simulink model "HubDepotModel_debug"  (Simulink 7.9)
settings: Solver=VariableStepDiscrete  StartTime=0.0  StopTime=100.0  RelTol=1e-3
libraries: simeventslib x2
settings Model: Creator=tsprock3  LastModifiedBy=tsprock3
settings DebuggingCC: SimStateOlderReleaseMsg=warning

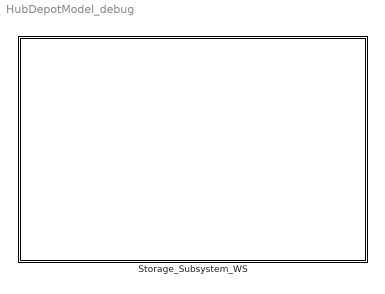
== system HubDepotModel_debug ==
  Storage_Subsystem_WS : Subsystem  AncestorBlock=DELS_Library/Storage_Subsystem_WS

== system HubDepotModel_debug/Storage_Subsystem_WS ==
  note: The Storage Subsystem mediates between the SOURCE and DELIVER channels, and provides higher levels control to those functions
  note: On the left hand side, customer procurement orders and replenishment shipments
      | come into the deliver and source functions respectively
  note: The processes associated with performing customer-facing order management and order fulfillment activities.
  note: The process of establishing and maintaining physical inventories and inventory information.
  note: The processes associated with ordering, delivery, receipt and transfer of raw material items, subassemblies, product and/or services.
  note: On the right hand side, procurement orders and fulfillment shipments
      | leave the source and deliver functions respectively
  note: The replenishment signal is primarily a mechanism for the reordering process to know that the inventory levels have
      | changed and that the inventory policy should be reviewed to determine if a procurement order is necessary. This is
      | effectively a continuous review policy
      |
      | There are other ways to accomplish this, and a periodic review policy is one such way.
  note: The INVENTORY IN/OUT is the passing of physical/electronic inventory records from their storage place in ENABLE
      |  to the functions that use the records to fulfill or procure inventory
  <<DELIVER>>Deliver_Stocked_Product : Subsystem
  <<ENABLE>> Manage_Product_Inventory : Subsystem
  <<SOURCE>> Source_Stocked_Product : Subsystem
  Customer_Procurement_Order : PMIOPort  Port=1  Side=Right
  Fulfillment_Shipment : PMIOPort  Port=2  Side=Right
  Procurement_Order : PMIOPort  Port=3  Side=Left
  Replenishment_Shipment : PMIOPort  Port=4  Side=Left
  connections:
  <<DELIVER>>Deliver_Stocked_Product/LConn2 -- Customer_Procurement_Order/RConn1
  <<DELIVER>>Deliver_Stocked_Product/RConn2 -- Fulfillment_Shipment/RConn1
  Replenishment_Shipment/RConn1 -- <<SOURCE>> Source_Stocked_Product/LConn2
  <<ENABLE>> Manage_Product_Inventory/LConn2 -- <<SOURCE>> Source_Stocked_Product/RConn1
  <<ENABLE>> Manage_Product_Inventory/RConn2 -- <<SOURCE>> Source_Stocked_Product/LConn1
  <<ENABLE>> Manage_Product_Inventory/LConn3 -- <<DELIVER>>Deliver_Stocked_Product/RConn3
  <<ENABLE>> Manage_Product_Inventory/RConn3 -- <<SOURCE>> Source_Stocked_Product/LConn3
  <<SOURCE>> Source_Stocked_Product/RConn2 -- Procurement_Order/RConn1
  <<DELIVER>>Deliver_Stocked_Product/RConn1 -- <<ENABLE>> Manage_Product_Inventory/LConn1
  <<DELIVER>>Deliver_Stocked_Product/LConn1 -- <<ENABLE>> Manage_Product_Inventory/RConn1

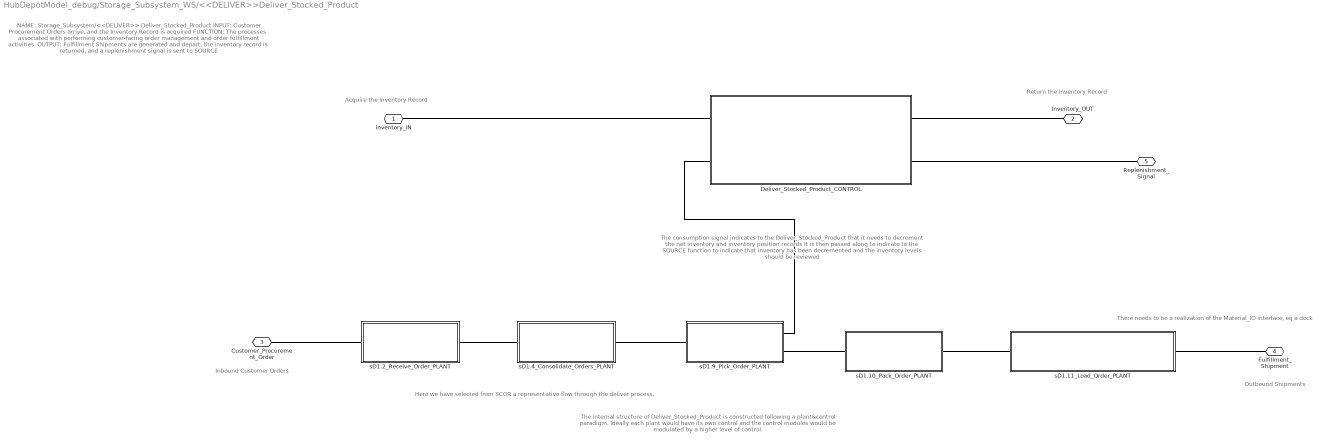
== system HubDepotModel_debug/Storage_Subsystem_WS/<<DELIVER>>Deliver_Stocked_Product ==
  note: The internal structure of Deliver_Stocked_Product is constructed following a plant&control paradigm. Ideally each plant would have its own control and the control modules would be modulated by a higher level of control.
  note: The consumption signal indicates to the Deliver_Stocked_Product that it needs to decrement the net inventory and inventory position records
      | It is then passed along to indicate to the SOURCE function to indicate that inventory has been decremented and the inventory levels should be reviewed
  note: Here we have selected from SCOR a representative flow through the deliver process.
  note: NAME: Storage_Subsystem/<<DELIVER>> Deliver_Stocked_Product
      | INPUT: Customer Procurement Orders arrive, and the Inventory Record is acquired
      | FUNCTION: The processes associated with performing customer-facing order management and order fulfillment activities.
      | OUTPUT: Fulfillment Shipments are generated and depart, the inventory record is returned, and a replenishment signal is sent to SOURCE
  note: Acquire the Inventory Record
  note: Return the Inventory Record
  note: Inbound Customer Orders
  note: Outbound Shipments
  note: There needs to be a realization of the Material_IO interface, eg a dock
  Deliver_Stocked_Product_CONTROL : Subsystem
  sD1.10_Pack_Order_PLANT : Subsystem
  sD1.11_Load_Order_PLANT : Subsystem
  sD1.2_Receive_Order_PLANT : Subsystem
  sD1.4_Consolidate_Orders_PLANT : Subsystem
  sD1.9_Pick_Order_PLANT : Subsystem
  Inventory_IN : PMIOPort  Port=1  Side=Left
  Inventory_OUT : PMIOPort  Port=2  Side=Right
  Customer_Procurement_Order : PMIOPort  Port=3  Side=Left
  Fulfillment_Shipment : PMIOPort  Port=4  Side=Right
  Replenishment_Signal : PMIOPort  Port=5  Side=Right
  connections:
  Customer_Procurement_Order/RConn1 -- sD1.2_Receive_Order_PLANT/LConn1
  sD1.9_Pick_Order_PLANT/RConn2 -- sD1.10_Pack_Order_PLANT/LConn1
  sD1.10_Pack_Order_PLANT/RConn1 -- sD1.11_Load_Order_PLANT/LConn1
  sD1.11_Load_Order_PLANT/RConn1 -- Fulfillment_Shipment/RConn1
  sD1.9_Pick_Order_PLANT/RConn1 -- Deliver_Stocked_Product_CONTROL/LConn2
  Deliver_Stocked_Product_CONTROL/LConn1 -- Inventory_IN/RConn1
  Deliver_Stocked_Product_CONTROL/RConn1 -- Inventory_OUT/RConn1
  sD1.2_Receive_Order_PLANT/RConn1 -- sD1.4_Consolidate_Orders_PLANT/LConn1
  sD1.4_Consolidate_Orders_PLANT/RConn1 -- sD1.9_Pick_Order_PLANT/LConn1
  Deliver_Stocked_Product_CONTROL/RConn2 -- Replenishment_Signal/RConn1

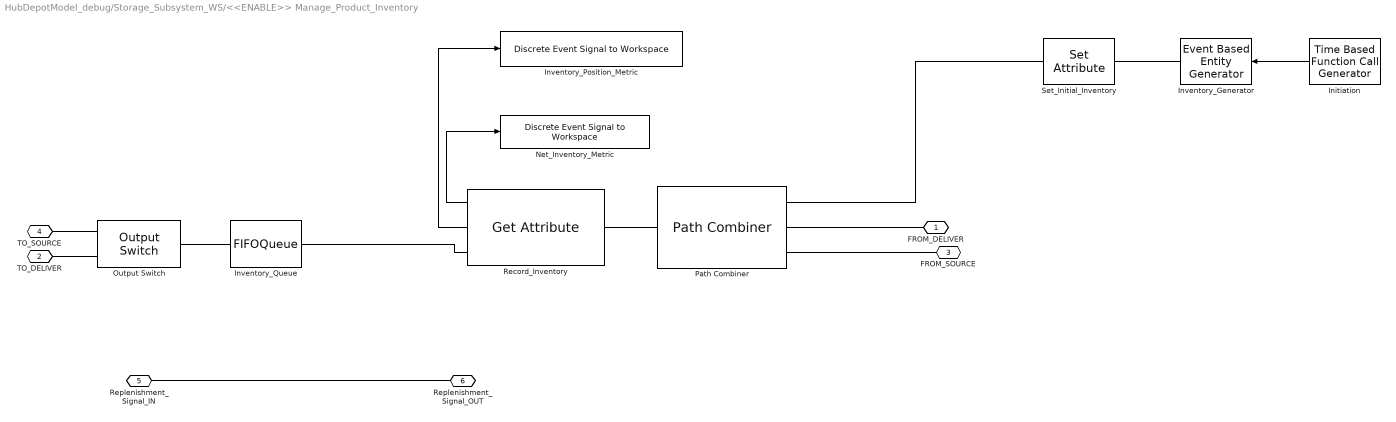
== system HubDepotModel_debug/Storage_Subsystem_WS/<<ENABLE>> Manage_Product_Inventory ==
  Initiation : TimeBasedFunctionCallGenerator  EventGenerationMode=Only at simulation start  EventPriority=1
  Inventory_Generator : EventBasedEntityGenerator  GenerateEntitiesUpon=Function call from port fcn  SpecifyEventPriority=on  PriorityEntityGeneration=1  AllowBlocking=off  EntityType=Standard
  Inventory_Position_Metric : simeventslib/SimEvents Sinks/Discrete Event Signal to Workspace  VariableName=Inventory_Position_Depot_1  SaveFormat=Structure With Time  isMonitorOnly=off  isRecordIC=off
  Inventory_Queue : FIFOQueue
  Net_Inventory_Metric : simeventslib/SimEvents Sinks/Discrete Event Signal to Workspace  VariableName=Net_Inventory_Depot_1  SaveFormat=Structure With Time  isMonitorOnly=off  isRecordIC=off
  Output Switch : OutputSwitch  NumberOutputPorts=2
  Path Combiner : PathCombiner
  Record_Inventory : GetAttribute  AttributeName=Net_Inventory|Inventory_Position  AttributeMissing=Error|Error  AttributeDefaultValue=1|1  AttributeTreatAsVector=1|1  AttributeSendTiming=After entity departure|After entity departure  EvaluatedDefaultAttributeValue={[];[]}
      settings: OutputPortMap=o1,o2
  Set_Initial_Inventory : SetAttribute  AttributeName=Net_Inventory|Inventory_Position|Reorder_Point|Reorder_Quantity  AttributeFrom=Dialog|Dialog|Dialog|Dialog  AttributeValue=InventoryParameters(:,1)|InventoryParameters(:,2)|InventoryParameters(:,3)|InventoryParameters(:,4)  AttributeTreatAsVector=1|1|1|1  EvaluatedAttributeValue={InventoryParameters(:,1);InventoryParameters(:,2);InventoryParameters(:,3);InventoryParameters(:,4)}
  FROM_DELIVER : PMIOPort  Port=1  Side=Left
  TO_DELIVER : PMIOPort  Port=2  Side=Right
  FROM_SOURCE : PMIOPort  Port=3  Side=Left
  TO_SOURCE : PMIOPort  Port=4  Side=Right
  Replenishment_Signal_IN : PMIOPort  Port=5  Side=Left
  Replenishment_Signal_OUT : PMIOPort  Port=6  Side=Right
  wires:
  Record_Inventory/1 -> Net_Inventory_Metric/1
  Initiation/1 -> Inventory_Generator/1
  Record_Inventory/2 -> Inventory_Position_Metric/1
  connections:
  Set_Initial_Inventory/LConn1 -- Inventory_Generator/RConn1
  Record_Inventory/RConn1 -- Inventory_Queue/LConn1
  Output Switch/LConn1 -- Inventory_Queue/RConn1
  Record_Inventory/LConn1 -- Path Combiner/RConn1
  FROM_DELIVER/RConn1 -- Path Combiner/LConn2
  FROM_SOURCE/RConn1 -- Path Combiner/LConn3
  TO_DELIVER/RConn1 -- Output Switch/RConn2
  TO_SOURCE/RConn1 -- Output Switch/RConn1
  Replenishment_Signal_IN/RConn1 -- Replenishment_Signal_OUT/RConn1
  Set_Initial_Inventory/RConn1 -- Path Combiner/LConn1

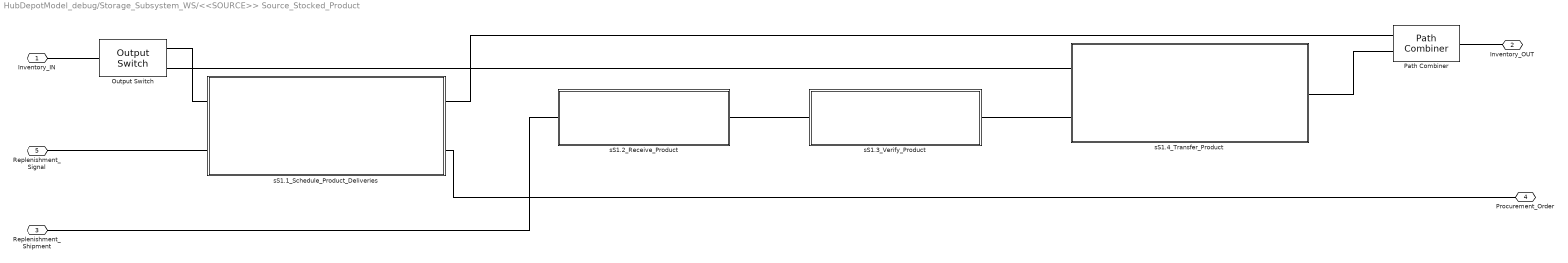
== system HubDepotModel_debug/Storage_Subsystem_WS/<<SOURCE>> Source_Stocked_Product ==
  Output Switch : OutputSwitch  NumberOutputPorts=2
  Path Combiner : PathCombiner  NumberInputPorts=2
  sS1.1_Schedule_Product_Deliveries : Subsystem
  sS1.2_Receive_Product : Subsystem
  sS1.3_Verify_Product : Subsystem
  sS1.4_Transfer_Product : Subsystem
  Inventory_IN : PMIOPort  Port=1  Side=Left
  Inventory_OUT : PMIOPort  Port=2  Side=Right
  Replenishment_Shipment : PMIOPort  Port=3  Side=Left
  Procurement_Order : PMIOPort  Port=4  Side=Right
  Replenishment_Signal : PMIOPort  Port=5  Side=Left
  connections:
  Output Switch/RConn1 -- sS1.1_Schedule_Product_Deliveries/LConn1
  sS1.1_Schedule_Product_Deliveries/RConn1 -- Path Combiner/LConn1
  Replenishment_Signal/RConn1 -- sS1.1_Schedule_Product_Deliveries/LConn2
  sS1.1_Schedule_Product_Deliveries/RConn2 -- Procurement_Order/RConn1
  sS1.4_Transfer_Product/RConn1 -- Path Combiner/LConn2
  Replenishment_Shipment/RConn1 -- sS1.2_Receive_Product/LConn1
  sS1.2_Receive_Product/RConn1 -- sS1.3_Verify_Product/LConn1
  sS1.3_Verify_Product/RConn1 -- sS1.4_Transfer_Product/LConn2
  Inventory_IN/RConn1 -- Output Switch/LConn1
  Output Switch/RConn2 -- sS1.4_Transfer_Product/LConn1
  Path Combiner/RConn1 -- Inventory_OUT/RConn1

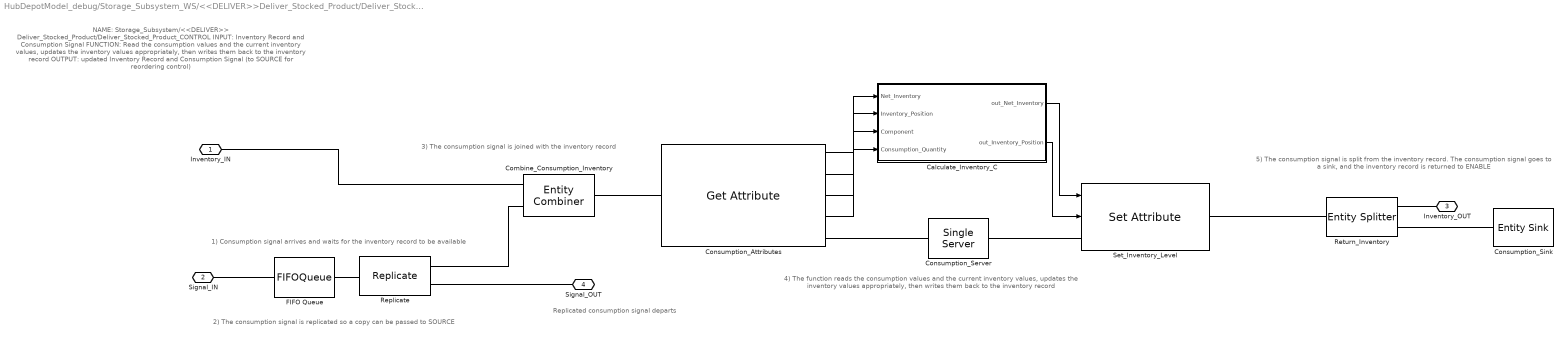
== system HubDepotModel_debug/Storage_Subsystem_WS/<<DELIVER>>Deliver_Stocked_Product/Deliver_Stocked_Product_CONTROL ==
  note: 1) Consumption signal arrives and waits for the inventory record to be available
  note: 2) The consumption signal is replicated so a copy can be passed to SOURCE
  note: Replicated consumption signal departs
  note: 3) The consumption signal is joined with the inventory record
  note: 4) The function reads the consumption values and the current inventory values, updates the inventory values appropriately,
      | then writes them back to the inventory record
  note: 5) The consumption signal is split from the inventory record.
      | The consumption signal goes to a sink, and the inventory record is returned to ENABLE
  note: NAME: Storage_Subsystem/<<DELIVER>> Deliver_Stocked_Product/Deliver_Stocked_Product_CONTROL
      | INPUT: Inventory Record and Consumption Signal
      | FUNCTION: Read the consumption values and the current inventory values, updates the inventory values appropriately, then writes them back to the inventory record
      | OUTPUT: updated Inventory Record and Consumption Signal (to SOURCE for reordering control)
  Calculate_Inventory_C : MATLAB Function  TreatAsAtomicUnit=on
  Combine_Consumption_Inventory : EntityCombiner  NumberInputPorts=2
  Consumption_Attributes : GetAttribute  AttributeName=Component|Consumption_Quantity|Net_Inventory|Inventory_Position  AttributeMissing=Error|Error|Error|Error  AttributeDefaultValue=1|1|1|1  AttributeTreatAsVector=1|1|1|1  AttributeSendTiming=After entity departure|After entity departure|After entity departure|After entity departure  EvaluatedDefaultAttributeValue={[];[];[];[]}
      settings: OutputPortMap=o1,o2,o3,o4
  Consumption_Server : SingleServer  ServiceTime=0
  Consumption_Sink : EntitySink
  FIFO Queue : FIFOQueue
  Replicate : Replicate  NumberOutputPorts=2
  Return_Inventory : EntitySplitter  NumberOutputPorts=2
  Set_Inventory_Level : SetAttribute  AttributeName=Net_Inventory|Inventory_Position  AttributeFrom=Signal port|Signal port  AttributeValue=1|1  AttributeTreatAsVector=1|1  EvaluatedAttributeValue={[];[]}
      settings: InputPortMap=u0,u1
  Inventory_IN : PMIOPort  Port=1  Side=Left
  Signal_IN : PMIOPort  Port=2  Side=Left
  Inventory_OUT : PMIOPort  Port=3  Side=Right
  Signal_OUT : PMIOPort  Port=4  Side=Right
  wires:
  Consumption_Attributes/1 -> Calculate_Inventory_C/3(Component)
  Calculate_Inventory_C/1(out_Net_Inventory) -> Set_Inventory_Level/1
  Consumption_Attributes/3 -> Calculate_Inventory_C/1(Net_Inventory)
  Consumption_Attributes/2 -> Calculate_Inventory_C/4(Consumption_Quantity)
  Consumption_Attributes/4 -> Calculate_Inventory_C/2(Inventory_Position)
  Calculate_Inventory_C/2(out_Inventory_Position) -> Set_Inventory_Level/2
  connections:
  Inventory_IN/RConn1 -- Combine_Consumption_Inventory/LConn1
  Replicate/RConn1 -- Combine_Consumption_Inventory/LConn2
  Combine_Consumption_Inventory/RConn1 -- Consumption_Attributes/LConn1
  Consumption_Attributes/RConn1 -- Consumption_Server/LConn1
  Consumption_Server/RConn1 -- Set_Inventory_Level/LConn1
  Return_Inventory/RConn2 -- Consumption_Sink/LConn1
  Replicate/RConn2 -- Signal_OUT/RConn1
  Set_Inventory_Level/RConn1 -- Return_Inventory/LConn1
  Inventory_OUT/RConn1 -- Return_Inventory/RConn1
  Signal_IN/RConn1 -- FIFO Queue/LConn1
  FIFO Queue/RConn1 -- Replicate/LConn1

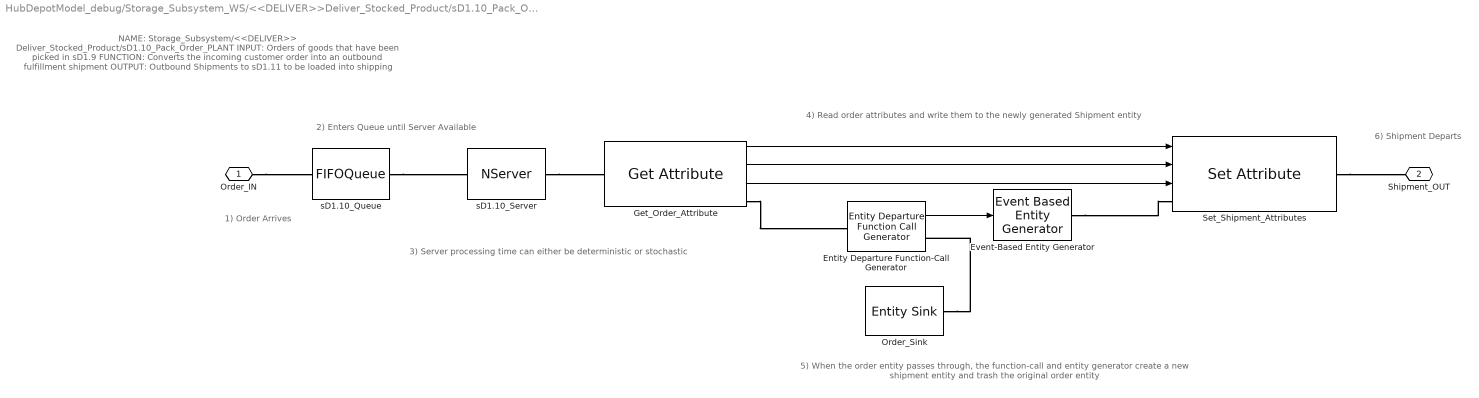
== system HubDepotModel_debug/Storage_Subsystem_WS/<<DELIVER>>Deliver_Stocked_Product/sD1.10_Pack_Order_PLANT ==
  note: NAME: Storage_Subsystem/<<DELIVER>> Deliver_Stocked_Product/sD1.10_Pack_Order_PLANT
      | INPUT: Orders of goods that have been picked in sD1.9
      | FUNCTION: Converts the incoming customer order into an outbound fulfillment shipment
      | OUTPUT: Outbound Shipments to sD1.11 to be loaded into shipping
  note: 1) Order Arrives
  note: 2) Enters Queue until Server Available
  note: 3) Server processing time can either be deterministic or stochastic
  note: 4) Read order attributes and write them to the newly generated Shipment entity
  note: 5) When the order entity passes through, the function-call and entity generator create a new shipment entity
      | and trash the original order entity
  note: 6) Shipment Departs
  Entity Departure Function-Call Generator : EntityDepartureFunctionCallGenerator
  Event-Based Entity Generator : EventBasedEntityGenerator  GenerateEntitiesUpon=Function call from port fcn
  Get_Order_Attribute : GetAttribute  AttributeName=Component|Order_Quantity|Customer  AttributeMissing=Error|Error|Error  AttributeDefaultValue=1|1|1  AttributeTreatAsVector=1|1|1  AttributeSendTiming=After entity departure|After entity departure|After entity departure  EvaluatedDefaultAttributeValue={[];[];[]}
      settings: OutputPortMap=o1,o2,o3
  Order_Sink : EntitySink
  Set_Shipment_Attributes : SetAttribute  AttributeName=Component|Shipment_Quantity|Customer  AttributeFrom=Signal port|Signal port|Signal port  AttributeValue=1|1|1  AttributeTreatAsVector=1|1|1  EvaluatedAttributeValue={[];[];[]}
      settings: InputPortMap=u0,u1,u2
  sD1.10_Queue : FIFOQueue
  sD1.10_Server : NServer  NumberOfServers=inf  ServiceTime=0
  Order_IN : PMIOPort  Port=1  Side=Left
  Shipment_OUT : PMIOPort  Port=2  Side=Right
  wires:
  Entity Departure Function-Call Generator/1 -> Event-Based Entity Generator/1
  Get_Order_Attribute/2 -> Set_Shipment_Attributes/2
  Get_Order_Attribute/1 -> Set_Shipment_Attributes/1
  Get_Order_Attribute/3 -> Set_Shipment_Attributes/3
  connections:
  sD1.10_Queue/RConn1 -- sD1.10_Server/LConn1
  Order_IN/RConn1 -- sD1.10_Queue/LConn1
  Event-Based Entity Generator/RConn1 -- Set_Shipment_Attributes/LConn1
  Set_Shipment_Attributes/RConn1 -- Shipment_OUT/RConn1
  Order_Sink/LConn1 -- Entity Departure Function-Call Generator/RConn1
  sD1.10_Server/RConn1 -- Get_Order_Attribute/LConn1
  Get_Order_Attribute/RConn1 -- Entity Departure Function-Call Generator/LConn1

== system HubDepotModel_debug/Storage_Subsystem_WS/<<DELIVER>>Deliver_Stocked_Product/sD1.11_Load_Order_PLANT ==
  sD1.11_Queue : FIFOQueue
  sD1.11_Server : NServer  NumberOfServers=inf  ServiceTime=0
  Shipment_IN : PMIOPort  Port=1  Side=Left
  Shipment_OUT : PMIOPort  Port=2  Side=Right
  connections:
  sD1.11_Queue/RConn1 -- sD1.11_Server/LConn1
  Shipment_IN/RConn1 -- sD1.11_Queue/LConn1
  Shipment_OUT/RConn1 -- sD1.11_Server/RConn1

== system HubDepotModel_debug/Storage_Subsystem_WS/<<DELIVER>>Deliver_Stocked_Product/sD1.2_Receive_Order_PLANT ==
  sD1.2_Queue : FIFOQueue
  sD1.2_Server : NServer  NumberOfServers=inf  ServiceTime=0
  Order_IN : PMIOPort  Port=1  Side=Left
  Order_OUT : PMIOPort  Port=2  Side=Right
  connections:
  sD1.2_Queue/RConn1 -- sD1.2_Server/LConn1
  Order_IN/RConn1 -- sD1.2_Queue/LConn1
  Order_OUT/RConn1 -- sD1.2_Server/RConn1

== system HubDepotModel_debug/Storage_Subsystem_WS/<<DELIVER>>Deliver_Stocked_Product/sD1.4_Consolidate_Orders_PLANT ==
  sD1.4_Queue : FIFOQueue
  sD1.4_Server : NServer  NumberOfServers=inf  ServiceTime=0
  Order_IN : PMIOPort  Port=1  Side=Left
  Order_OUT : PMIOPort  Port=2  Side=Right
  connections:
  sD1.4_Queue/RConn1 -- sD1.4_Server/LConn1
  Order_IN/RConn1 -- sD1.4_Queue/LConn1
  Order_OUT/RConn1 -- sD1.4_Server/RConn1

== system HubDepotModel_debug/Storage_Subsystem_WS/<<DELIVER>>Deliver_Stocked_Product/sD1.9_Pick_Order_PLANT ==
  Generate_Consumption_Signal : Subsystem
  sD1.9_Queue : FIFOQueue
  sD1.9_Server : NServer  NumberOfServers=inf  ServiceTime=0
  Order_IN : PMIOPort  Port=1  Side=Left
  Signal_OUT : PMIOPort  Port=2  Side=Right
  Order_OUT : PMIOPort  Port=3  Side=Right
  connections:
  sD1.9_Queue/RConn1 -- sD1.9_Server/LConn1
  Order_IN/RConn1 -- sD1.9_Queue/LConn1
  sD1.9_Server/RConn1 -- Generate_Consumption_Signal/LConn1
  Generate_Consumption_Signal/RConn1 -- Order_OUT/RConn1
  Generate_Consumption_Signal/RConn2 -- Signal_OUT/RConn1

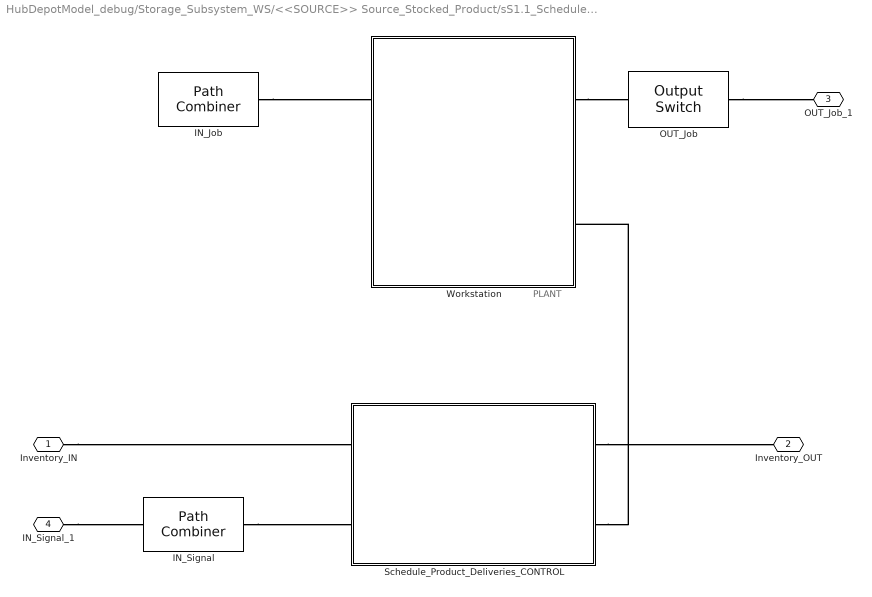
== system HubDepotModel_debug/Storage_Subsystem_WS/<<SOURCE>> Source_Stocked_Product/sS1.1_Schedule_Product_Deliveries ==
  note: PLANT
  IN_Job : PathCombiner  NumberInputPorts=1
  IN_Signal : PathCombiner  NumberInputPorts=1
  OUT_Job : OutputSwitch  NumberOutputPorts=1
  Schedule_Product_Deliveries_CONTROL : Subsystem
  Workstation : Subsystem
  Inventory_IN : PMIOPort  Port=1  Side=Left
  Inventory_OUT : PMIOPort  Port=2  Side=Right
  OUT_Job_1 : PMIOPort  Port=3  Side=Right
  IN_Signal_1 : PMIOPort  Port=4  Side=Left
  connections:
  IN_Signal_1/RConn1 -- IN_Signal/LConn1
  IN_Signal/RConn1 -- Schedule_Product_Deliveries_CONTROL/LConn2
  Workstation/RConn1 -- OUT_Job/LConn1
  OUT_Job/RConn1 -- OUT_Job_1/RConn1
  Schedule_Product_Deliveries_CONTROL/RConn2 -- Workstation/RConn2
  Schedule_Product_Deliveries_CONTROL/RConn1 -- Inventory_OUT/RConn1
  Inventory_IN/RConn1 -- Schedule_Product_Deliveries_CONTROL/LConn1
  IN_Job/RConn1 -- Workstation/LConn1

== system HubDepotModel_debug/Storage_Subsystem_WS/<<SOURCE>> Source_Stocked_Product/sS1.2_Receive_Product ==
  note: PLANT
  IN_Job : PathCombiner  NumberInputPorts=1
  OUT_Job : OutputSwitch  NumberOutputPorts=1
  Receive_Product_CONTROL : Subsystem
  Workstation : Subsystem
  IN_Job_1 : PMIOPort  Port=1  Side=Left
  OUT_Job_1 : PMIOPort  Port=2  Side=Right
  connections:
  OUT_Job/RConn1 -- OUT_Job_1/RConn1
  Workstation/RConn1 -- OUT_Job/LConn1
  Receive_Product_CONTROL/RConn1 -- Workstation/RConn2
  IN_Job_1/RConn1 -- IN_Job/LConn1
  Workstation/LConn2 -- Receive_Product_CONTROL/LConn1
  IN_Job/RConn1 -- Workstation/LConn1

== system HubDepotModel_debug/Storage_Subsystem_WS/<<SOURCE>> Source_Stocked_Product/sS1.3_Verify_Product ==
  note: PLANT
  IN_Job : PathCombiner  NumberInputPorts=1
  OUT_Job : OutputSwitch  NumberOutputPorts=1
  Verify_Product_CONTROL : Subsystem
  Workstation : Subsystem
  IN_Job_1 : PMIOPort  Port=1  Side=Left
  OUT_Job_1 : PMIOPort  Port=2  Side=Right
  connections:
  OUT_Job/RConn1 -- OUT_Job_1/RConn1
  Workstation/RConn1 -- OUT_Job/LConn1
  Verify_Product_CONTROL/RConn1 -- Workstation/RConn2
  IN_Job_1/RConn1 -- IN_Job/LConn1
  Workstation/LConn2 -- Verify_Product_CONTROL/LConn1
  IN_Job/RConn1 -- Workstation/LConn1

== system HubDepotModel_debug/Storage_Subsystem_WS/<<SOURCE>> Source_Stocked_Product/sS1.4_Transfer_Product ==
  note: PLANT
  IN_Job : PathCombiner  NumberInputPorts=1
  Transfer_Product_CONTROL : Subsystem
  Workstation : Subsystem
  Inventory_IN : PMIOPort  Port=1  Side=Left
  IN_Job_1 : PMIOPort  Port=2  Side=Left
  Inventory_OUT : PMIOPort  Port=3  Side=Right
  connections:
  Transfer_Product_CONTROL/RConn2 -- Workstation/RConn2
  Transfer_Product_CONTROL/RConn1 -- Inventory_OUT/RConn1
  Inventory_IN/RConn1 -- Transfer_Product_CONTROL/LConn1
  IN_Job_1/RConn1 -- IN_Job/LConn1
  Workstation/LConn2 -- Transfer_Product_CONTROL/LConn2
  IN_Job/RConn1 -- Workstation/LConn1

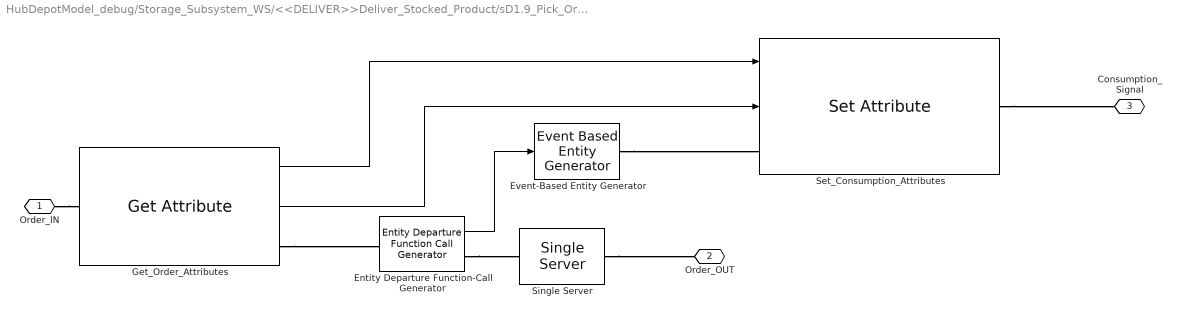
== system HubDepotModel_debug/Storage_Subsystem_WS/<<DELIVER>>Deliver_Stocked_Product/sD1.9_Pick_Order_PLANT/Generate_Consumption_Signal ==
  Entity Departure Function-Call Generator : EntityDepartureFunctionCallGenerator
  Event-Based Entity Generator : EventBasedEntityGenerator  GenerateEntitiesUpon=Function call from port fcn
  Get_Order_Attributes : GetAttribute  AttributeName=Component|Order_Quantity  AttributeMissing=Error|Error  AttributeDefaultValue=1|1  AttributeTreatAsVector=1|1  AttributeSendTiming=After entity departure|After entity departure  EvaluatedDefaultAttributeValue={[];[]}
      settings: OutputPortMap=o1,o2
  Set_Consumption_Attributes : SetAttribute  AttributeName=Component|Consumption_Quantity  AttributeFrom=Signal port|Signal port  AttributeValue=1|1  AttributeTreatAsVector=1|1  EvaluatedAttributeValue={[];[]}
      settings: InputPortMap=u0,u1
  Single Server : SingleServer  ServiceTime=0
  Order_IN : PMIOPort  Port=1  Side=Left
  Order_OUT : PMIOPort  Port=2  Side=Right
  Consumption_Signal : PMIOPort  Port=3  Side=Right
  wires:
  Entity Departure Function-Call Generator/1 -> Event-Based Entity Generator/1
  Get_Order_Attributes/1 -> Set_Consumption_Attributes/1
  Get_Order_Attributes/2 -> Set_Consumption_Attributes/2
  connections:
  Single Server/RConn1 -- Order_OUT/RConn1
  Entity Departure Function-Call Generator/RConn1 -- Single Server/LConn1
  Get_Order_Attributes/RConn1 -- Entity Departure Function-Call Generator/LConn1
  Event-Based Entity Generator/RConn1 -- Set_Consumption_Attributes/LConn1
  Set_Consumption_Attributes/RConn1 -- Consumption_Signal/RConn1
  Order_IN/RConn1 -- Get_Order_Attributes/LConn1

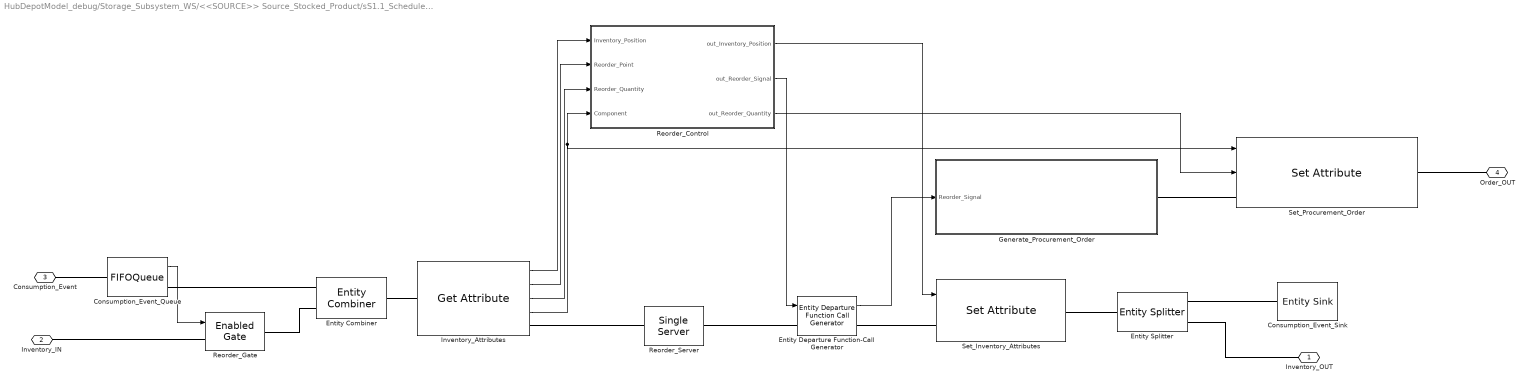
== system HubDepotModel_debug/Storage_Subsystem_WS/<<SOURCE>> Source_Stocked_Product/sS1.1_Schedule_Product_Deliveries/Schedule_Product_Deliveries_CONTROL ==
  Consumption_Event_Queue : FIFOQueue  StatNumberInBlock=on
      settings: OutputPortMap=o1
  Consumption_Event_Sink : EntitySink
  Entity Combiner : EntityCombiner  NumberInputPorts=2
  Entity Departure Function-Call Generator : EntityDepartureFunctionCallGenerator  EnableE1Port=on
  Entity Splitter : EntitySplitter  NumberOutputPorts=2
  Generate_Procurement_Order : Subsystem
  Inventory_Attributes : GetAttribute  AttributeName=Inventory_Position|Reorder_Point|Reorder_Quantity|Component  AttributeMissing=Error|Error|Error|Error  AttributeDefaultValue=1|1|1|1  AttributeTreatAsVector=1|1|1|1  AttributeSendTiming=After entity departure|After entity departure|After entity departure|After entity departure  EvaluatedDefaultAttributeValue={[];[];[];[]}
      settings: OutputPortMap=o1,o2,o3,o4
  Reorder_Control : MATLAB Function  TreatAsAtomicUnit=on
  Reorder_Gate : EnabledGate  SpecifyEventPriority=on  PriorityGateEnableOpenClose=1
  Reorder_Server : SingleServer  ServiceTime=0
  Set_Inventory_Attributes : SetAttribute  AttributeName=Inventory_Position  AttributeFrom=Signal port  EvaluatedAttributeValue={[]}
  Set_Procurement_Order : SetAttribute  AttributeName=Component|Order_Quantity|Supplier|Customer  AttributeFrom=Signal port|Signal port|Dialog|Dialog  AttributeValue=1|1|1|1  AttributeTreatAsVector=1|1|1|1  EvaluatedAttributeValue={[];[];1;1}
      settings: InputPortMap=u0,u1
  Inventory_OUT : PMIOPort  Port=1  Side=Right
  Inventory_IN : PMIOPort  Port=2  Side=Left
  Consumption_Event : PMIOPort  Port=3  Side=Left
  Order_OUT : PMIOPort  Port=4  Side=Right
  wires:
  Consumption_Event_Queue/1 -> Reorder_Gate/1
  Reorder_Control/3(out_Reorder_Quantity) -> Set_Procurement_Order/2
  Reorder_Control/1(out_Inventory_Position) -> Set_Inventory_Attributes/1
  Reorder_Control/2(out_Reorder_Signal) -> Entity Departure Function-Call Generator/1
  Entity Departure Function-Call Generator/1 -> Generate_Procurement_Order/1(Reorder_Signal)
  Inventory_Attributes/1 -> Reorder_Control/1(Inventory_Position)
  Inventory_Attributes/2 -> Reorder_Control/2(Reorder_Point)
  Inventory_Attributes/3 -> Reorder_Control/3(Reorder_Quantity)
  Inventory_Attributes/4 -> Reorder_Control/4(Component), Set_Procurement_Order/1
  connections:
  Inventory_IN/RConn1 -- Reorder_Gate/LConn1
  Inventory_Attributes/RConn1 -- Reorder_Server/LConn1
  Entity Combiner/RConn1 -- Inventory_Attributes/LConn1
  Reorder_Gate/RConn1 -- Entity Combiner/LConn2
  Entity Splitter/RConn1 -- Consumption_Event_Sink/LConn1
  Consumption_Event_Queue/RConn1 -- Entity Combiner/LConn1
  Consumption_Event/RConn1 -- Consumption_Event_Queue/LConn1
  Set_Inventory_Attributes/RConn1 -- Entity Splitter/LConn1
  Generate_Procurement_Order/RConn1 -- Set_Procurement_Order/LConn1
  Reorder_Server/RConn1 -- Entity Departure Function-Call Generator/LConn1
  Entity Departure Function-Call Generator/RConn1 -- Set_Inventory_Attributes/LConn1
  Entity Splitter/RConn2 -- Inventory_OUT/RConn1
  Set_Procurement_Order/RConn1 -- Order_OUT/RConn1

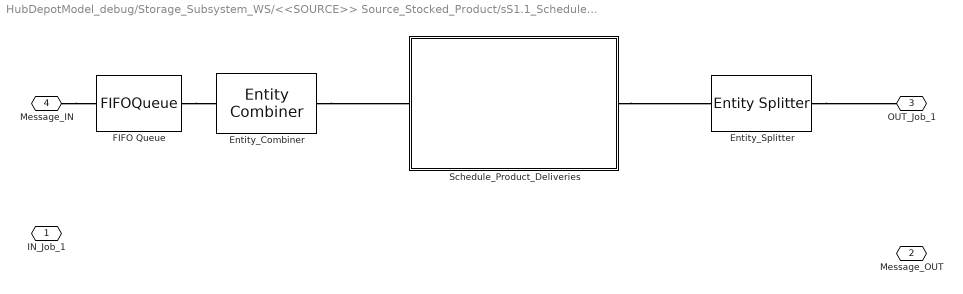
== system HubDepotModel_debug/Storage_Subsystem_WS/<<SOURCE>> Source_Stocked_Product/sS1.1_Schedule_Product_Deliveries/Workstation ==
  Entity_Combiner : EntityCombiner  NumberInputPorts=1
  Entity_Splitter : EntitySplitter  NumberOutputPorts=1
  FIFO Queue : FIFOQueue
  Schedule_Product_Deliveries : Subsystem
  IN_Job_1 : PMIOPort  Port=1  Side=Left
  Message_OUT : PMIOPort  Port=2  Side=Left
  OUT_Job_1 : PMIOPort  Port=3  Side=Right
  Message_IN : PMIOPort  Port=4  Side=Right
  connections:
  Entity_Splitter/RConn1 -- OUT_Job_1/RConn1
  Message_IN/RConn1 -- FIFO Queue/LConn1
  Schedule_Product_Deliveries/RConn1 -- Entity_Splitter/LConn1
  Entity_Combiner/RConn1 -- Schedule_Product_Deliveries/LConn1
  FIFO Queue/RConn1 -- Entity_Combiner/LConn1

== system HubDepotModel_debug/Storage_Subsystem_WS/<<SOURCE>> Source_Stocked_Product/sS1.2_Receive_Product/Receive_Product_CONTROL ==
  Message_IN : PMIOPort  Port=1  Side=Left
  Message_OUT : PMIOPort  Port=2  Side=Right
  connections:
  Message_IN/RConn1 -- Message_OUT/RConn1

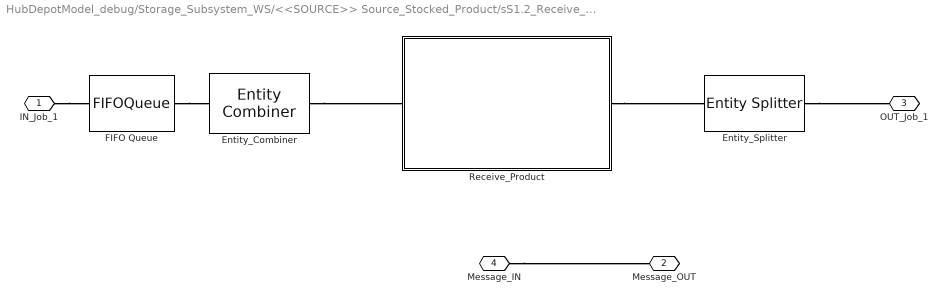
== system HubDepotModel_debug/Storage_Subsystem_WS/<<SOURCE>> Source_Stocked_Product/sS1.2_Receive_Product/Workstation ==
  Entity_Combiner : EntityCombiner  NumberInputPorts=1
  Entity_Splitter : EntitySplitter  NumberOutputPorts=1
  FIFO Queue : FIFOQueue
  Receive_Product : Subsystem
  IN_Job_1 : PMIOPort  Port=1  Side=Left
  Message_OUT : PMIOPort  Port=2  Side=Left
  OUT_Job_1 : PMIOPort  Port=3  Side=Right
  Message_IN : PMIOPort  Port=4  Side=Right
  connections:
  Entity_Splitter/RConn1 -- OUT_Job_1/RConn1
  Message_IN/RConn1 -- Message_OUT/RConn1
  Receive_Product/RConn1 -- Entity_Splitter/LConn1
  Entity_Combiner/RConn1 -- Receive_Product/LConn1
  IN_Job_1/RConn1 -- FIFO Queue/LConn1
  FIFO Queue/RConn1 -- Entity_Combiner/LConn1

== system HubDepotModel_debug/Storage_Subsystem_WS/<<SOURCE>> Source_Stocked_Product/sS1.3_Verify_Product/Verify_Product_CONTROL ==
  Message_IN : PMIOPort  Port=1  Side=Left
  Message_OUT : PMIOPort  Port=2  Side=Right
  connections:
  Message_IN/RConn1 -- Message_OUT/RConn1

== system HubDepotModel_debug/Storage_Subsystem_WS/<<SOURCE>> Source_Stocked_Product/sS1.3_Verify_Product/Workstation ==
  Entity_Combiner : EntityCombiner  NumberInputPorts=1
  Entity_Splitter : EntitySplitter  NumberOutputPorts=1
  FIFO Queue : FIFOQueue
  Verify_Product : Subsystem
  IN_Job_1 : PMIOPort  Port=1  Side=Left
  Message_OUT : PMIOPort  Port=2  Side=Left
  OUT_Job_1 : PMIOPort  Port=3  Side=Right
  Message_IN : PMIOPort  Port=4  Side=Right
  connections:
  Entity_Splitter/RConn1 -- OUT_Job_1/RConn1
  Message_IN/RConn1 -- Message_OUT/RConn1
  Verify_Product/RConn1 -- Entity_Splitter/LConn1
  Entity_Combiner/RConn1 -- Verify_Product/LConn1
  IN_Job_1/RConn1 -- FIFO Queue/LConn1
  FIFO Queue/RConn1 -- Entity_Combiner/LConn1

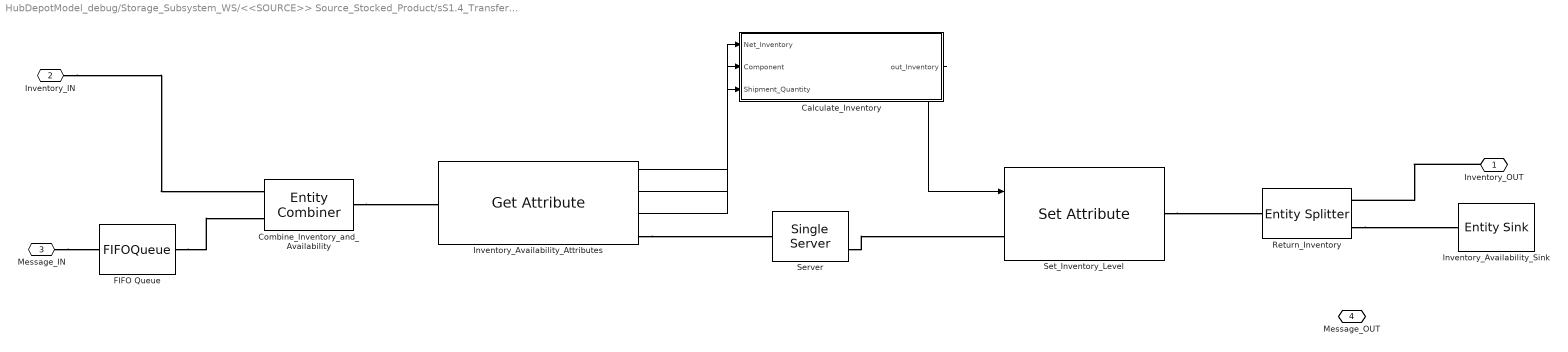
== system HubDepotModel_debug/Storage_Subsystem_WS/<<SOURCE>> Source_Stocked_Product/sS1.4_Transfer_Product/Transfer_Product_CONTROL ==
  Calculate_Inventory : MATLAB Function  TreatAsAtomicUnit=on
  Combine_Inventory_and_Availability : EntityCombiner  NumberInputPorts=2
  FIFO Queue : FIFOQueue
  Inventory_Availability_Attributes : GetAttribute  AttributeName=Component|Shipment_Quantity|Net_Inventory  AttributeMissing=Error|Error|Error  AttributeDefaultValue=1|1|1  AttributeTreatAsVector=1|1|1  AttributeSendTiming=After entity departure|After entity departure|After entity departure  EvaluatedDefaultAttributeValue={[];[];[]}
      settings: OutputPortMap=o1,o2,o3
  Inventory_Availability_Sink : EntitySink
  Return_Inventory : EntitySplitter  NumberOutputPorts=2
  Server : SingleServer  ServiceTime=0  StatNumberDeparted=on
  Set_Inventory_Level : SetAttribute  AttributeName=Net_Inventory  AttributeFrom=Signal port  EvaluatedAttributeValue={[]}
  Inventory_OUT : PMIOPort  Port=1  Side=Right
  Inventory_IN : PMIOPort  Port=2  Side=Left
  Message_IN : PMIOPort  Port=3  Side=Left
  Message_OUT : PMIOPort  Port=4  Side=Right
  wires:
  Inventory_Availability_Attributes/2 -> Calculate_Inventory/3(Shipment_Quantity)
  Inventory_Availability_Attributes/3 -> Calculate_Inventory/1(Net_Inventory)
  Calculate_Inventory/1(out_Inventory) -> Set_Inventory_Level/1
  Inventory_Availability_Attributes/1 -> Calculate_Inventory/2(Component)
  connections:
  Inventory_IN/RConn1 -- Combine_Inventory_and_Availability/LConn1
  FIFO Queue/RConn1 -- Combine_Inventory_and_Availability/LConn2
  Message_IN/RConn1 -- FIFO Queue/LConn1
  Inventory_OUT/RConn1 -- Return_Inventory/RConn1
  Set_Inventory_Level/RConn1 -- Return_Inventory/LConn1
  Return_Inventory/RConn2 -- Inventory_Availability_Sink/LConn1
  Server/RConn1 -- Set_Inventory_Level/LConn1
  Inventory_Availability_Attributes/RConn1 -- Server/LConn1
  Combine_Inventory_and_Availability/RConn1 -- Inventory_Availability_Attributes/LConn1

== system HubDepotModel_debug/Storage_Subsystem_WS/<<SOURCE>> Source_Stocked_Product/sS1.4_Transfer_Product/Workstation ==
  note: Inventory Availability Signal
  Entity_Combiner : EntityCombiner  NumberInputPorts=1
  Entity_Splitter : EntitySplitter  NumberOutputPorts=1
  FIFO Queue : FIFOQueue
  Transfer_Product : Subsystem
  IN_Job_1 : PMIOPort  Port=1  Side=Left
  Message_OUT : PMIOPort  Port=2  Side=Left
  OUT_Job_1 : PMIOPort  Port=3  Side=Right
  Message_IN : PMIOPort  Port=4  Side=Right
  connections:
  Entity_Splitter/RConn1 -- Message_OUT/RConn1
  Transfer_Product/RConn1 -- Entity_Splitter/LConn1
  Entity_Combiner/RConn1 -- Transfer_Product/LConn1
  IN_Job_1/RConn1 -- FIFO Queue/LConn1
  FIFO Queue/RConn1 -- Entity_Combiner/LConn1

== system HubDepotModel_debug/Storage_Subsystem_WS/<<SOURCE>> Source_Stocked_Product/sS1.1_Schedule_Product_Deliveries/Schedule_Product_Deliveries_CONTROL/Generate_Procurement_Order ==
  Reorder_Signal : Inport
  Event-Based Entity Generator : EventBasedEntityGenerator  GenerateEntitiesUpon=Function call from port fcn
  Blank_Procurement_Order : PMIOPort  Port=1  Side=Right
  wires:
  Reorder_Signal/1 -> Event-Based Entity Generator/1
  connections:
  Blank_Procurement_Order/RConn1 -- Event-Based Entity Generator/RConn1

== system HubDepotModel_debug/Storage_Subsystem_WS/<<SOURCE>> Source_Stocked_Product/sS1.1_Schedule_Product_Deliveries/Workstation/Schedule_Product_Deliveries ==
  IN_Job : PathCombiner  NumberInputPorts=1
  OUT_Job : OutputSwitch  NumberOutputPorts=1  SwitchingCriterion=Equiprobable
  Process : Subsystem
  IN_Job_1 : PMIOPort  Port=1  Side=Left
  OUT_Job_1 : PMIOPort  Port=2  Side=Right
  connections:
  OUT_Job/RConn1 -- OUT_Job_1/RConn1
  IN_Job_1/RConn1 -- IN_Job/LConn1
  Process/RConn1 -- OUT_Job/LConn1
  IN_Job/RConn1 -- Process/LConn1

== system HubDepotModel_debug/Storage_Subsystem_WS/<<SOURCE>> Source_Stocked_Product/sS1.2_Receive_Product/Workstation/Receive_Product ==
  IN_Job : PathCombiner  NumberInputPorts=1
  OUT_Job : OutputSwitch  NumberOutputPorts=1  SwitchingCriterion=Equiprobable
  Process : Subsystem
  IN_Job_1 : PMIOPort  Port=1  Side=Left
  OUT_Job_1 : PMIOPort  Port=2  Side=Right
  connections:
  OUT_Job/RConn1 -- OUT_Job_1/RConn1
  IN_Job_1/RConn1 -- IN_Job/LConn1
  Process/RConn1 -- OUT_Job/LConn1
  IN_Job/RConn1 -- Process/LConn1

== system HubDepotModel_debug/Storage_Subsystem_WS/<<SOURCE>> Source_Stocked_Product/sS1.3_Verify_Product/Workstation/Verify_Product ==
  IN_Job : PathCombiner  NumberInputPorts=1
  OUT_Job : OutputSwitch  NumberOutputPorts=1  SwitchingCriterion=Equiprobable
  Process : Subsystem
  IN_Job_1 : PMIOPort  Port=1  Side=Left
  OUT_Job_1 : PMIOPort  Port=2  Side=Right
  connections:
  OUT_Job/RConn1 -- OUT_Job_1/RConn1
  IN_Job_1/RConn1 -- IN_Job/LConn1
  Process/RConn1 -- OUT_Job/LConn1
  IN_Job/RConn1 -- Process/LConn1

== system HubDepotModel_debug/Storage_Subsystem_WS/<<SOURCE>> Source_Stocked_Product/sS1.4_Transfer_Product/Workstation/Transfer_Product ==
  IN_Job : PathCombiner  NumberInputPorts=1
  OUT_Job : OutputSwitch  NumberOutputPorts=1  SwitchingCriterion=Equiprobable
  Process : Subsystem
  IN_Job_1 : PMIOPort  Port=1  Side=Left
  OUT_Job_1 : PMIOPort  Port=2  Side=Right
  connections:
  OUT_Job/RConn1 -- OUT_Job_1/RConn1
  IN_Job_1/RConn1 -- IN_Job/LConn1
  Process/RConn1 -- OUT_Job/LConn1
  IN_Job/RConn1 -- Process/LConn1

== system HubDepotModel_debug/Storage_Subsystem_WS/<<SOURCE>> Source_Stocked_Product/sS1.1_Schedule_Product_Deliveries/Workstation/Schedule_Product_Deliveries/Process ==
  FIFO Queue : FIFOQueue  Capacity=inf
  N-Server : NServer  NumberOfServers=inf  ServiceTimeFrom=Signal port t
  ProcessTime : EventBasedRandomNumber  Distribution=Gaussian (normal)  minUnif=1  meanNorm=5
  Job_OUT : PMIOPort  Port=1  Side=Right
  Job_IN : PMIOPort  Port=2  Side=Left
  wires:
  ProcessTime/1 -> N-Server/1
  connections:
  Job_IN/RConn1 -- FIFO Queue/LConn1
  Job_OUT/RConn1 -- N-Server/RConn1
  FIFO Queue/RConn1 -- N-Server/LConn1

== system HubDepotModel_debug/Storage_Subsystem_WS/<<SOURCE>> Source_Stocked_Product/sS1.2_Receive_Product/Workstation/Receive_Product/Process ==
  FIFO Queue : FIFOQueue  Capacity=inf
  N-Server : NServer  NumberOfServers=inf  ServiceTimeFrom=Signal port t
  ProcessTime : EventBasedRandomNumber  Distribution=Gaussian (normal)  minUnif=1  meanNorm=5
  Job_OUT : PMIOPort  Port=1  Side=Right
  Job_IN : PMIOPort  Port=2  Side=Left
  wires:
  ProcessTime/1 -> N-Server/1
  connections:
  Job_IN/RConn1 -- FIFO Queue/LConn1
  Job_OUT/RConn1 -- N-Server/RConn1
  FIFO Queue/RConn1 -- N-Server/LConn1

== system HubDepotModel_debug/Storage_Subsystem_WS/<<SOURCE>> Source_Stocked_Product/sS1.3_Verify_Product/Workstation/Verify_Product/Process ==
  FIFO Queue : FIFOQueue  Capacity=inf
  N-Server : NServer  NumberOfServers=inf  ServiceTimeFrom=Signal port t
  ProcessTime : EventBasedRandomNumber  Distribution=Gaussian (normal)  minUnif=1  meanNorm=5
  Job_OUT : PMIOPort  Port=1  Side=Right
  Job_IN : PMIOPort  Port=2  Side=Left
  wires:
  ProcessTime/1 -> N-Server/1
  connections:
  Job_IN/RConn1 -- FIFO Queue/LConn1
  Job_OUT/RConn1 -- N-Server/RConn1
  FIFO Queue/RConn1 -- N-Server/LConn1

== system HubDepotModel_debug/Storage_Subsystem_WS/<<SOURCE>> Source_Stocked_Product/sS1.4_Transfer_Product/Workstation/Transfer_Product/Process ==
  FIFO Queue : FIFOQueue  Capacity=inf
  N-Server : NServer  NumberOfServers=inf  ServiceTimeFrom=Signal port t
  ProcessTime : EventBasedRandomNumber  Distribution=Gaussian (normal)  minUnif=1  meanNorm=5
  Job_OUT : PMIOPort  Port=1  Side=Right
  Job_IN : PMIOPort  Port=2  Side=Left
  wires:
  ProcessTime/1 -> N-Server/1
  connections:
  Job_IN/RConn1 -- FIFO Queue/LConn1
  Job_OUT/RConn1 -- N-Server/RConn1
  FIFO Queue/RConn1 -- N-Server/LConn1

== matlab function Storage_Subsystem_WS/<<DELIVER>>Deliver_Stocked_Product/Deliver_Stocked_Product_CONTROL/Calculate_Inventory_C ==
  data: Net_Inventory input double; Inventory_Position input double; out_Net_Inventory output double; Component input double; Consumption_Quantity input double; out_Inventory_Position output double
function [out_Net_Inventory,out_Inventory_Position] = fcn(Net_Inventory, Inventory_Position, Component, Consumption_Quantity)
%#codegen

%coder.extrinsic('str2num');

%y = zeros(1, 'int32');
%y = Type;
out_Net_Inventory = Net_Inventory;
out_Inventory_Position = Inventory_Position;
if eq(Component, 0) == 0
    out_Net_Inventory(Component) = Net_Inventory(Component) - Consumption_Quantity;
    out_Inventory_Position(Component) = Inventory_Position(Component) - Consumption_Quantity;
end

end

== matlab function Storage_Subsystem_WS/<<SOURCE>> Source_Stocked_Product/sS1.1_Schedule_Product_Deliveries/Schedule_Product_Deliveries_CONTROL/Reorder_Control ==
  data: Inventory_Position input double; Reorder_Point input double; Reorder_Quantity input double; Component input double; out_Inventory_Position output double; out_Reorder_Signal output double; out_Reorder_Quantity output double
function [out_Inventory_Position, out_Reorder_Signal, out_Reorder_Quantity] = fcn(Inventory_Position, Reorder_Point, Reorder_Quantity, Component)
%This function is a combination of all the CONTROL systems at once

out_Inventory_Position = Inventory_Position;
out_Reorder_Signal =0;
out_Reorder_Quantity = 0;
if eq(Component, 0) == 0
    %Operative Subsystem Control
    if Inventory_Position(Component) <= Reorder_Point(Component)
        out_Reorder_Signal = Reorder_Quantity(Component);
        out_Reorder_Quantity = Reorder_Quantity(Component);
        
        %Control & Monitoring Subsystem
        out_Inventory_Position(Component) = Inventory_Position(Component) + Reorder_Quantity(Component);
        
    end
end

== matlab function Storage_Subsystem_WS/<<SOURCE>> Source_Stocked_Product/sS1.4_Transfer_Product/Transfer_Product_CONTROL/Calculate_Inventory ==
  data: Net_Inventory input double; out_Inventory output double; Component input double; Shipment_Quantity input double
function out_Inventory = fcn(Net_Inventory, Component, Shipment_Quantity)
%#codegen

%coder.extrinsic('str2num');

%y = zeros(1, 'int32');
%y = Type;
out_Inventory = Net_Inventory;
if eq(Component, 0) == 0
    out_Inventory(Component) = Net_Inventory(Component) + Shipment_Quantity;
end

end
